simulink model "Excercise1and2"  (R2019b)
settings: Solver=VariableStepAuto  StartTime=0.0  StopTime=20  RelTol=1e-3
values from neighbouring files (symbols this model uses):
  CD = -2    [NewtonsSecondLaw.m]
  gc = -32.2    [NewtonsSecondLaw.m]
  m = mlbm / gc    (= -3.16770186335)    [NewtonsSecondLaw.m]
settings Model: Creator=dzecc  LastModifiedBy=dzecc

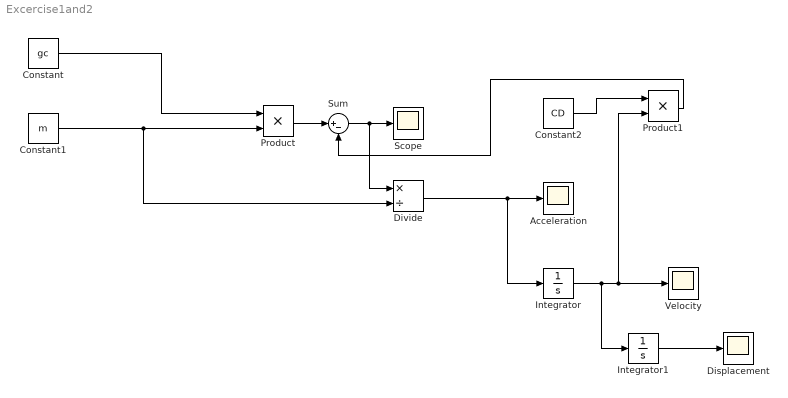
== system Excercise1and2 ==
  Acceleration : Scope
  Constant : Constant  Value=gc  SampleTime=10
  Constant1 : Constant  Value=m  SampleTime=10
  Constant2 : Constant  Value=CD  SampleTime=10
  Displacement : Scope
  Divide : Product  Inputs=*/
  Integrator : Integrator  InitialCondition=200
  Integrator1 : Integrator  InitialCondition=1
  Product : Product
  Product1 : Product
  Scope : Scope
  Sum : Sum  Inputs=|+-
  Velocity : Scope
  wires:
  Constant/1 -> Product/1
  Divide/1 -> Integrator/1, Acceleration/1
  Integrator/1 -> Integrator1/1, Product1/2, Velocity/1
  Integrator1/1 -> Displacement/1
  Sum/1 -> Divide/1, Scope/1
  Constant1/1 -> Divide/2, Product/2
  Product/1 -> Sum/1
  Product1/1 -> Sum/2
  Constant2/1 -> Product1/1
